simulink model "PHIL_SupportFunctions"  (R2016a)
settings: Solver=FixedStepDiscrete  StartTime=0.0  StopTime=15  FixedStep=1e-2  RelTol=1e-3
settings Model: Creator=CoSES_HPC2  LastModifiedBy=CoSES_HPC2
settings DebuggingCC: RootOutportRequireBusObject=error  StrictBusMsg=ErrorOnBusTreatedAsVector
settings HardwareCC: ProdBitPerPointer=32  ProdLargestAtomicFloat=None  ProdWordSize=32  ProdHWDeviceType=Intel->x86/Pentium
settings RTWCC: SystemTargetFile=NIVeriStand.tlc  TemplateMakefile=NIVeriStand_vc.tmf  Description=NI Phar Lap Real-Time & Windows Targets
settings STFCustomTargetCC: MatFileLogging=on  SystemTargetFile=NIVeriStand.tlc
settings GRTTargetCC: ParMdlRefBuildCompliant=off  CompOptLevelCompliant=off  ConcurrentExecutionCompliant=off  GeneratePreprocessorConditionals=Use local settings  CombineOutputUpdateFcns=off  CPPClassGenCompliant=off  GRTInterface=on  UseToolchainInfoCompliant=off

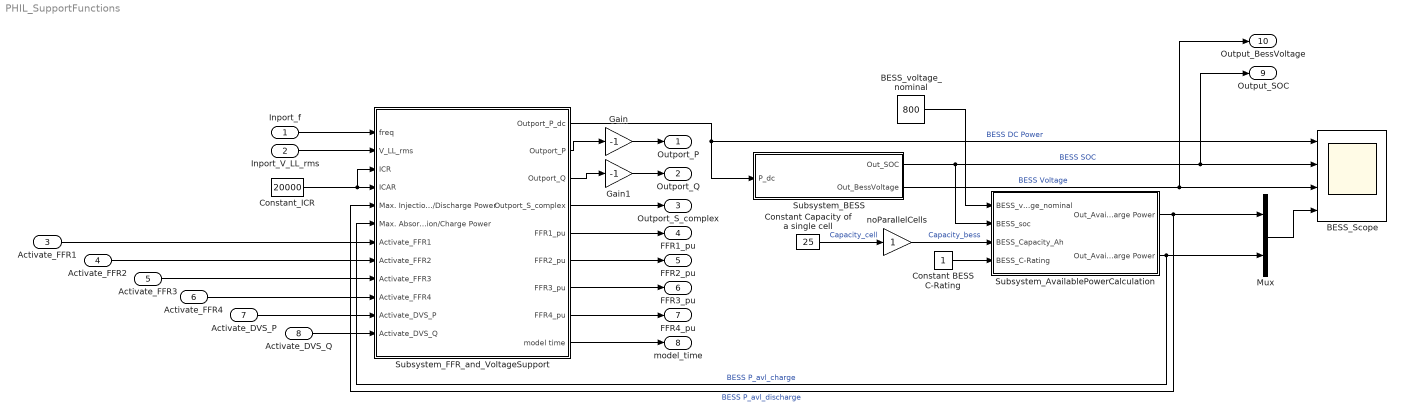
== system PHIL_SupportFunctions ==
  Inport_f : Inport
  Inport_V_LL_rms : Inport  Port=2
  Activate_FFR1 : Inport  Port=3
  Activate_FFR2 : Inport  Port=4
  Activate_FFR3 : Inport  Port=5
  Activate_FFR4 : Inport  Port=6
  Activate_DVS_P : Inport  Port=7
  Activate_DVS_Q : Inport  Port=8
  BESS_Scope : Scope  NumInputPorts=4
  BESS_voltage_nominal : Constant  Value=800
  Constant BESS C-Rating : Constant
  Constant Capacity of a single cell : Constant  Value=25
  Constant_ICR : Constant  Value=20000
  Gain : Gain  Gain=-1
  Gain1 : Gain  Gain=-1
  Mux : Mux  Inputs=2
  Subsystem_AvailablePowerCalculation : Subsystem
  Subsystem_BESS : Subsystem
  Subsystem_FFR_and_VoltageSupport : Subsystem
  noParallelCells : Gain
  Outport_P : Outport
  Outport_Q : Outport  Port=2
  Outport_S_complex : Outport  Port=3
  FFR1_pu : Outport  Port=4
  FFR2_pu : Outport  Port=5
  FFR3_pu : Outport  Port=6
  FFR4_pu : Outport  Port=7
  model_time : Outport  Port=8
  Output_SOC : Outport  Port=9
  Output_BessVoltage : Outport  Port=10
  wires:
  Constant_ICR/1 -> Subsystem_FFR_and_VoltageSupport/3(ICR), Subsystem_FFR_and_VoltageSupport/4(ICAR)
  Subsystem_AvailablePowerCalculation/2(Out_Available Charge Power) -> Subsystem_FFR_and_VoltageSupport/6(Max. Absorption/Charge Power), Mux/2  "BESS P_avl_charge"
  noParallelCells/1 -> Subsystem_AvailablePowerCalculation/3(BESS_Capacity_Ah)  "Capacity_bess"
  Subsystem_BESS/2(Out_BessVoltage) -> Output_BessVoltage/1, BESS_Scope/3  "BESS Voltage"
  Constant BESS C-Rating/1 -> Subsystem_AvailablePowerCalculation/4(BESS_C-Rating)
  Mux/1 -> BESS_Scope/4
  Subsystem_AvailablePowerCalculation/1(Out_Available Discharge Power) -> Subsystem_FFR_and_VoltageSupport/5(Max. Injection/Discharge Power), Mux/1  "BESS P_avl_discharge"
  Subsystem_BESS/1(Out_SOC) -> Output_SOC/1, BESS_Scope/2, Subsystem_AvailablePowerCalculation/2(BESS_soc)  "BESS SOC"
  BESS_voltage_nominal/1 -> Subsystem_AvailablePowerCalculation/1(BESS_voltage_nominal)
  Constant Capacity of a single cell/1 -> noParallelCells/1  "Capacity_cell"
  Subsystem_FFR_and_VoltageSupport/1(Outport_P_dc) -> BESS_Scope/1, Subsystem_BESS/1(P_dc)  "BESS DC Power"
  Subsystem_FFR_and_VoltageSupport/8(FFR4_pu) -> FFR4_pu/1
  Subsystem_FFR_and_VoltageSupport/7(FFR3_pu) -> FFR3_pu/1
  Subsystem_FFR_and_VoltageSupport/6(FFR2_pu) -> FFR2_pu/1
  Subsystem_FFR_and_VoltageSupport/5(FFR1_pu) -> FFR1_pu/1
  Subsystem_FFR_and_VoltageSupport/4(Outport_S_complex) -> Outport_S_complex/1
  Inport_V_LL_rms/1 -> Subsystem_FFR_and_VoltageSupport/2(V_LL_rms)
  Inport_f/1 -> Subsystem_FFR_and_VoltageSupport/1(freq)
  Subsystem_FFR_and_VoltageSupport/9(model time) -> model_time/1
  Gain/1 -> Outport_P/1
  Subsystem_FFR_and_VoltageSupport/2(Outport_P) -> Gain/1
  Gain1/1 -> Outport_Q/1
  Subsystem_FFR_and_VoltageSupport/3(Outport_Q) -> Gain1/1
  Activate_FFR1/1 -> Subsystem_FFR_and_VoltageSupport/7(Activate_FFR1)
  Activate_FFR2/1 -> Subsystem_FFR_and_VoltageSupport/8(Activate_FFR2)
  Activate_FFR3/1 -> Subsystem_FFR_and_VoltageSupport/9(Activate_FFR3)
  Activate_FFR4/1 -> Subsystem_FFR_and_VoltageSupport/10(Activate_FFR4)
  Activate_DVS_P/1 -> Subsystem_FFR_and_VoltageSupport/11(Activate_DVS_P)
  Activate_DVS_Q/1 -> Subsystem_FFR_and_VoltageSupport/12(Activate_DVS_Q)

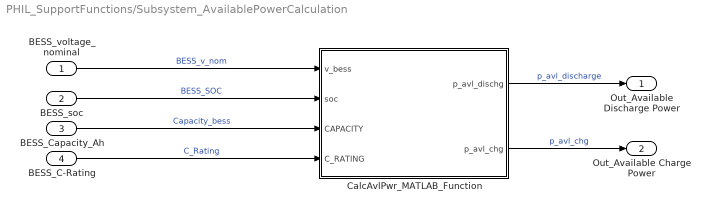
== system PHIL_SupportFunctions/Subsystem_AvailablePowerCalculation ==
  BESS_voltage_nominal : Inport
  BESS_soc : Inport  Port=2
  BESS_Capacity_Ah : Inport  Port=3
  BESS_C-Rating : Inport  Port=4
  CalcAvlPwr_MATLAB_Function : MATLAB Function  TreatAsAtomicUnit=on
  Out_Available Discharge Power : Outport
  Out_Available Charge Power : Outport  Port=2
  wires:
  CalcAvlPwr_MATLAB_Function/1(p_avl_dischg) -> Out_Available Discharge Power/1  "p_avl_discharge"
  BESS_voltage_nominal/1 -> CalcAvlPwr_MATLAB_Function/1(v_bess)  "BESS_v_nom"
  BESS_Capacity_Ah/1 -> CalcAvlPwr_MATLAB_Function/3(CAPACITY)  "Capacity_bess"
  CalcAvlPwr_MATLAB_Function/2(p_avl_chg) -> Out_Available Charge Power/1  "p_avl_chg"
  BESS_soc/1 -> CalcAvlPwr_MATLAB_Function/2(soc)  "BESS_SOC"
  BESS_C-Rating/1 -> CalcAvlPwr_MATLAB_Function/4(C_RATING)  "C_Rating"

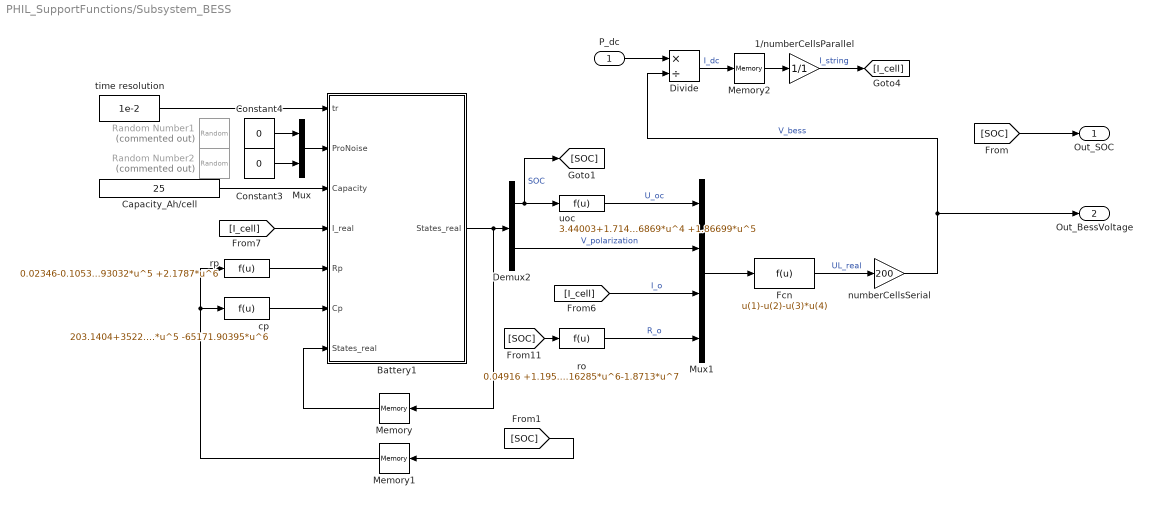
== system PHIL_SupportFunctions/Subsystem_BESS ==
  P_dc : Inport
  1/numberCellsParallel : Gain  Gain=1/1
  Battery1 : MATLAB Function  TreatAsAtomicUnit=on
  Capacity_Ah/cell : Constant  Value=25
  Constant3 : Constant  Value=0
  Constant4 : Constant  Value=0
  Demux2 : Demux  Outputs=2
  Divide : Product  Inputs=*/
  Fcn : Fcn  Expr=u(1)-u(2)-u(3)*u(4)
  Memory : Memory  X0=[0.6;0]  LinearizeAsDelay=on
  Memory1 : Memory  X0=0.6  LinearizeAsDelay=on
  Memory2 : Memory
  Mux : Mux  Inputs=2
  Mux1 : Mux
  Random Number1 : RandomNumber  Commented=on  Variance=2e-8  SampleTime=5e-4
  Random Number2 : RandomNumber  Commented=on  Variance=1e-8  SampleTime=5e-4
  cp : Fcn  Expr=203.1404+3522.78847*u-31392.66753*u^2+122406.91269*u^3-227590.94382*u^4+198281.56406*u^5 -65171.90395*u^6
  numberCellsSerial : Gain  Gain=200
  ro : Fcn  Expr=0.04916 +1.19552*u-6.25333*u^2+14.24181*u^3-13.93388*u^4+2.553*u^5+4.16285*u^6-1.8713*u^7
  rp : Fcn  Expr=0.02346-0.10537*u^1+1.1371*u^2-4.55188*u^3+8.26827*u^4-6.93032*u^5 +2.1787*u^6
  time resolution : Constant  Value=1e-2
  uoc : Fcn  Expr=3.44003+1.71448*u -3.51247*u^2 +5.70868*u^3 -5.06869*u^4 +1.86699*u^5
  Out_SOC : Outport
  Out_BessVoltage : Outport  Port=2
  wires:
  Mux/1 -> Battery1/2(ProNoise)
  Fcn/1 -> numberCellsSerial/1  "UL_real"
  Memory1/1 -> cp/1, rp/1
  time resolution/1 -> Battery1/1(tr)
  Memory/1 -> Battery1/7("States_real ")
  ro/1 -> Mux1/4  "R_o"
  uoc/1 -> Mux1/1  "U_oc"
  Demux2/1 -> [SOC], uoc/1  "SOC"
  Demux2/2 -> Mux1/2  "V_polarization"
  Mux1/1 -> Fcn/1
  Constant3/1 -> Mux/2
  Constant4/1 -> Mux/1
  [I_cell] -> Mux1/3  "I_o"
  Battery1/1(States_real) -> Memory/1, Demux2/1
  rp/1 -> Battery1/5(Rp)
  cp/1 -> Battery1/6(Cp)
  Capacity_Ah/cell/1 -> Battery1/3(Capacity)
  P_dc/1 -> Divide/1
  Divide/1 -> Memory2/1  "I_dc"
  Memory2/1 -> 1/numberCellsParallel/1
  [I_cell] -> Battery1/4(I_real)
  1/numberCellsParallel/1 -> [I_cell]  "I_string"
  numberCellsSerial/1 -> Divide/2, Out_BessVoltage/1  "V_bess"
  [SOC] -> Out_SOC/1
  [SOC] -> Memory1/1
  [SOC] -> ro/1

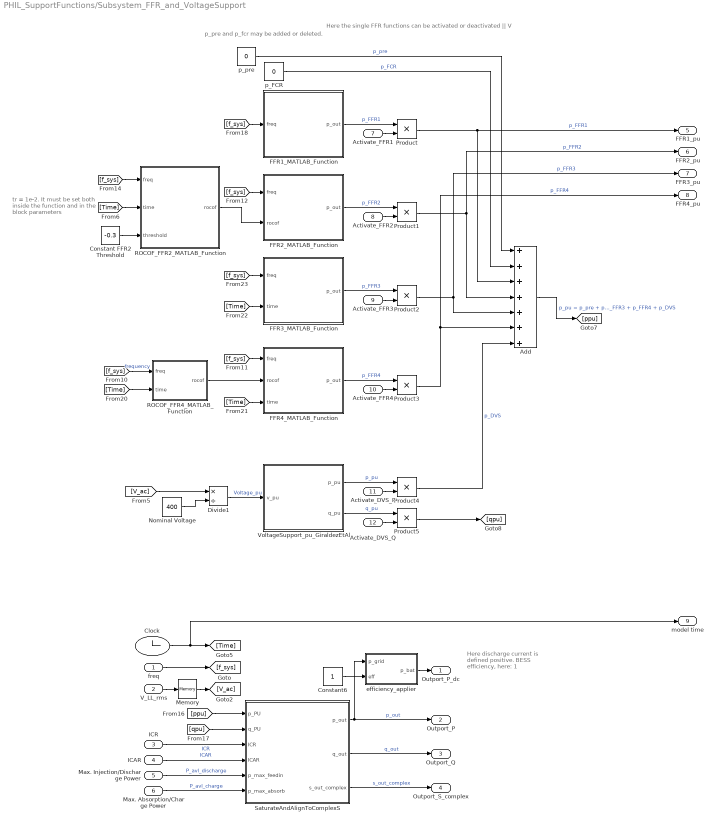
== system PHIL_SupportFunctions/Subsystem_FFR_and_VoltageSupport ==
  note: tr = 1e-2. It must be set
      | both inside the function
      | and in the block parameters
  note: Here discharge
      | current is defined positive.
      | BESS efficiency, here: 1
  note: Here the single FFR functions can be activated or deactivated
      |                                                ||
      |                                                V
  note: p_pre and p_fcr may be added or deleted.
  freq : Inport
  V_LL_rms : Inport  Port=2
  ICR : Inport  Port=3
  ICAR : Inport  Port=4
  Max. Injection/Discharge Power : Inport  Port=5
  Max. Absorption/Charge Power : Inport  Port=6
  Activate_FFR1 : Inport  Port=7
  Activate_FFR2 : Inport  Port=8
  Activate_FFR3 : Inport  Port=9
  Activate_FFR4 : Inport  Port=10
  Activate_DVS_P : Inport  Port=11
  Activate_DVS_Q : Inport  Port=12
  Add : Sum  Inputs=+++++++
  Clock : Clock
  Constant FFR2 Threshold : Constant  Value=-0.3
  Constant6 : Constant
  Divide1 : Product  Inputs=*/
  FFR1_MATLAB_Function : MATLAB Function  TreatAsAtomicUnit=on  SystemSampleTime=1e-2
  FFR2_MATLAB_Function : MATLAB Function  TreatAsAtomicUnit=on  SystemSampleTime=1e-2
  FFR3_MATLAB_Function : MATLAB Function  TreatAsAtomicUnit=on  SystemSampleTime=1e-2
  FFR4_MATLAB_Function : MATLAB Function  TreatAsAtomicUnit=on  SystemSampleTime=1e-2
  Memory : Memory  X0=400
  Nominal Voltage : Constant  Value=400
  Product{,1..5} (6 alike) : Product
  ROCOF_FFR2_MATLAB_Function : MATLAB Function  TreatAsAtomicUnit=on  SystemSampleTime=1e-2
  ROCOF_FFR4_MATLAB_Function : MATLAB Function  TreatAsAtomicUnit=on  SystemSampleTime=1e-2
  SaturateAndAlignToComplexS : MATLAB Function  TreatAsAtomicUnit=on
  VoltageSupport_pu_GiraldezEtAl : MATLAB Function  TreatAsAtomicUnit=on
  efficiency_applier : MATLAB Function  TreatAsAtomicUnit=on
  p_FCR : Constant  Value=0
  p_pre : Constant  Value=0
  Outport_P_dc : Outport
  Outport_P : Outport  Port=2
  Outport_Q : Outport  Port=3
  Outport_S_complex : Outport  Port=4
  FFR1_pu : Outport  Port=5
  FFR2_pu : Outport  Port=6
  FFR3_pu : Outport  Port=7
  FFR4_pu : Outport  Port=8
  model time : Outport  Port=9
  wires:
  efficiency_applier/1(p_bat) -> Outport_P_dc/1
  freq/1 -> [f_sys]
  Max. Injection/Discharge Power/1 -> SaturateAndAlignToComplexS/5(p_max_feedin)  "P_avl_discharge"
  Nominal Voltage/1 -> Divide1/2
  Divide1/1 -> VoltageSupport_pu_GiraldezEtAl/1(v_pu)  "Voltage_pu"
  Max. Absorption/Charge Power/1 -> SaturateAndAlignToComplexS/6(p_max_absorb)  "P_avl_charge"
  SaturateAndAlignToComplexS/2(q_out) -> Outport_Q/1  "q_out"
  SaturateAndAlignToComplexS/3(s_out_complex) -> Outport_S_complex/1  "s_out_complex"
  Memory/1 -> [V_ac]
  [ppu] -> SaturateAndAlignToComplexS/1(p_PU)
  [qpu] -> SaturateAndAlignToComplexS/2(q_PU)
  SaturateAndAlignToComplexS/1(p_out) -> efficiency_applier/1(p_grid), Outport_P/1  "p_out"
  ICR/1 -> SaturateAndAlignToComplexS/3(ICR)  "ICR"
  ICAR/1 -> SaturateAndAlignToComplexS/4(ICAR)  "ICAR"
  Product5/1 -> [qpu]
  Product/1 -> Add/3, FFR1_pu/1  "p_FFR1"
  ROCOF_FFR4_MATLAB_Function/1(rocof) -> FFR4_MATLAB_Function/2(rocof)
  FFR2_MATLAB_Function/1(p_out) -> Product1/1  "p_FFR2"
  ROCOF_FFR2_MATLAB_Function/1(rocof) -> FFR2_MATLAB_Function/2(rocof)
  p_FCR/1 -> Add/2  "p_FCR"
  Product3/1 -> FFR4_pu/1, Add/6  "p_FFR4"
  [f_sys] -> FFR3_MATLAB_Function/1(freq)
  FFR1_MATLAB_Function/1(p_out) -> Product/1  "p_FFR1"
  p_pre/1 -> Add/1  "p_pre"
  FFR4_MATLAB_Function/1(p_out) -> Product3/1  "p_FFR4"
  [f_sys] -> FFR2_MATLAB_Function/1(freq)
  FFR3_MATLAB_Function/1(p_out) -> Product2/1  "p_FFR3"
  [f_sys] -> ROCOF_FFR2_MATLAB_Function/1(freq)
  [Time] -> FFR3_MATLAB_Function/2(time)
  Constant FFR2 Threshold/1 -> ROCOF_FFR2_MATLAB_Function/3(threshold)
  Product1/1 -> Add/4, FFR2_pu/1  "p_FFR2"
  Product2/1 -> FFR3_pu/1, Add/5  "p_FFR3"
  Clock/1 -> model time/1, [Time]
  [f_sys] -> ROCOF_FFR4_MATLAB_Function/1(freq)  "frequency"
  [f_sys] -> FFR4_MATLAB_Function/1(freq)
  [Time] -> FFR4_MATLAB_Function/3(time)
  [Time] -> ROCOF_FFR4_MATLAB_Function/2(time)
  [f_sys] -> FFR1_MATLAB_Function/1(freq)
  [Time] -> ROCOF_FFR2_MATLAB_Function/2(time)
  Product4/1 -> Add/7  "p_DVS"
  Add/1 -> [ppu]  "p_pu = p_pre + p_FFR1 + p_FFR2 + p_FFR3 + p_FFR4 + p_DVS"
  VoltageSupport_pu_GiraldezEtAl/2(q_pu) -> Product5/1  "q_pu"
  VoltageSupport_pu_GiraldezEtAl/1(p_pu) -> Product4/1  "p_pu"
  V_LL_rms/1 -> Memory/1
  Activate_FFR1/1 -> Product/2
  Activate_FFR3/1 -> Product2/2
  Activate_FFR2/1 -> Product1/2
  Activate_FFR4/1 -> Product3/2
  Activate_DVS_P/1 -> Product4/2
  Activate_DVS_Q/1 -> Product5/2
  [V_ac] -> Divide1/1
  Constant6/1 -> efficiency_applier/2(eff)

== matlab function PHIL_SupportFunctions/Subsystem_FFR_and_VoltageSupport/SaturateAndAlignToComplexS ==
  data: p_out output; q_out output; p_PU input; q_PU input; s_out_complex output; ICR input; ICAR input; p_max_feedin input; p_max_absorb input
% This function computes the complex power reference for the converter from
% the p.u. values of active and reactive power, respectively, as well as
% the maximum converter power and the maximum available BESS power.
%
% Active power is defined as positive when supplying energy to the grid (=discharging the BESS)
%
%##### Input description #####
% p_PU         : active power reference (in p.u.)
% q_PU         : reactive power reference (in p.u.)
% ICR          : Maximum Converter Power (in VA) (ICR = IBR continuous rating, IBR = Inverter-Based Resources)
% ICAR         : Maximum Converter Power for absorption (in VA) (ICAR = IBR continuous absorption rating)
% p_max_feedin : Maximum available Power from BESS for feedin / discharge BESS (in W)
% p_max_absorb : Maximum available Power from BESS for absorption / charge BESS (in W)
%##### Output description #####
% p_out        : Active Power Reference (in W)
% q_out        : Reactive Power Reference (in var)
% s_out_complex: Complex Power Reference (in VA)

function [p_out,q_out,s_out_complex]  = ComplexApparentPower(p_PU, q_PU, ICR, ICAR, p_max_feedin, p_max_absorb)
% ISR in Watt (ISR = IBR short-term rating) may be added

% Reactive Power
q_out = q_PU*ICR; % q_PU is already saturated to +-0.44, hence no further treatment necessary

% Active Power
if p_PU >= 1              % positive active power, Saturation and Limiting to maximum grid injection / BESS discharge power
    p_out = p_max_feedin; 
elseif p_PU > 0           % positive active power, linear FFR range
    p_out = p_PU * p_max_feedin;
elseif p_PU <= -1         % negative active power, Saturation and Limiting to maximum grid absorption / BESS charge power
    p_out = -abs(p_max_absorb); 
elseif p_PU < 0           % negative active power, linear Voltage support range
    p_out = p_PU * abs(p_max_absorb); % (p_pu is already negative, so multiply with a positive number)
else % p_PU == 0          % zero output power
    p_out = 0;
end

% Complex Power
s_out_complex = complex(p_out,q_out); 
if p_out < 0
    if abs(s_out_complex) > ICAR
        p_out = -sqrt((ICAR^2)-(q_out^2));
    end
else % p_out >= 0
    if abs(s_out_complex) > ICR
        p_out = sqrt((ICR^2)-(q_out^2));
    end
end
    s_out_complex = complex(p_out,q_out); 
end

== matlab function PHIL_SupportFunctions/Subsystem_FFR_and_VoltageSupport/VoltageSupport_pu_GiraldezEtAl ==
  data: v_pu input; p_pu output; q_pu output
% This function computes the active and reactive output power in p.u. from
% the measured grid voltage in p.u. according to [Giraldez et al.]

function [p_pu,q_pu] = VoltageSupport(v_pu)

Q_max = 0.44; % in p.u.

if v_pu >= 0.97 && v_pu <= 1.03
    p_pu = 0;
    q_pu = 0;
elseif v_pu > 1.03
    if v_pu < 1.06
        p_pu = 0;
        q_pu = (1.03-v_pu)*(Q_max/0.03);
    elseif v_pu < 1.1
        p_pu = (1.06-v_pu)*(1/0.04);
        q_pu = -Q_max;
    else % v_pu >= 1.1
        p_pu = -1;
        q_pu = -Q_max;
    end
else % v_pu < 0.97
    p_pu = 0;
    if v_pu > 0.94
        q_pu = (0.97-v_pu)*(Q_max/0.03);
    else % v_pu <= 0.94
        q_pu = Q_max;
    end
end
end

== matlab function PHIL_SupportFunctions/Subsystem_AvailablePowerCalculation/CalcAvlPwr_MATLAB_Function ==
  data: v_bess input; p_avl_dischg output; soc input; CAPACITY input; p_avl_chg output; C_RATING input
% This function computes the Battery Energy Storage's (BESS') 
% available power for both the discharging and charging case.
% 
%##### Input description #####
% v_bess  : Voltage (V) of the BESS
% soc     : State of Charge (p.u. (1 means full)) of the BESS
% CAPACITY: Capacity (Ah) of the BESS
% C_RATING: C-Rating (p.u.) of the BESS = of the cells
%##### Output description #####
% p_avl_dischg: maximum available discharge power (W) 
% p_avl_chg   : maximum available charge power (W)

function [p_avl_dischg,p_avl_chg] = CalcAvailablePwr(v_bess, soc, CAPACITY, C_RATING) 
%% Constants Definition
DERATING_START_AT_SOC = 0.3;    % Assuming linear derating from SOC=30% downwards and from 70% upwards
P_MAX = C_RATING * CAPACITY * v_bess;  % Maximum BESS power, w/o consideration of SOC.

%% Algorithm for Calculation of available Discharge Power
if soc > DERATING_START_AT_SOC
    p_avl_dischg = P_MAX;
elseif soc > 0
    p_avl_dischg = P_MAX * soc / DERATING_START_AT_SOC;
else 
    p_avl_dischg = 0;
end

%% Algorithm for Calculation of available Charge Power
if soc < (1-DERATING_START_AT_SOC)
    p_avl_chg = P_MAX;
elseif soc < 1
    p_avl_chg = P_MAX * (1-soc) / DERATING_START_AT_SOC;
else
    p_avl_chg = 0;
end
end

== matlab function PHIL_SupportFunctions/Subsystem_FFR_and_VoltageSupport/FFR1_MATLAB_Function ==
  data: freq input; p_out output
% This function computes the FFR_1 power output in p.u. based on the
% current measured or observed frequency handed over in Hz. 

function p_out = FFR_1(freq)

fnom = 50;       % 50 Hz
fUF_FFR1 = 49.9; % Minimum: 99.17% of fnom, Maximum: 99.94% of fnom, Default: 99.94% of fnom [IEEE Std 2800-2022], Here: 99.8% of fnom
kUF_FFR1 = 0.01; % Minimum: 1%, Maximum: 5%, Default: 1% [IEEE Std 2800-2022]

if freq<fUF_FFR1
    p_out = (fUF_FFR1 - freq)/(fnom*kUF_FFR1);
else
    p_out = 0;
end
end

== matlab function PHIL_SupportFunctions/Subsystem_FFR_and_VoltageSupport/FFR2_MATLAB_Function ==
  data: freq input; p_out output; rocof input
% This function computes the FFR_2 power output in p.u. based on the
% current frequency in Hz and rate of change of frequency (RoCoF) in Hz/s, 
% both handed over as transfer parameters.

function p_out = FFR_2(freq, rocof)

fnom = 50;       % 50 Hz (here just informative)
fUF_FFR2 = 49.7; % Min: 99.17% of fnom, Max: N/A, Default: 99.4% of fnom (used here) [IEEE Std 2800-2022]
kUF_FFR2 = 0.5;  % Min: 0, Max: 5, Default: 0.5 [IEEE Std 2800-2022], (Here: 2.5)

if freq>fUF_FFR2 % idle, i.e. NOT triggered
    p_out = 0;
else % triggered, i.e. freq <= fUF_FFR2
    p_out = -kUF_FFR2 * rocof;
end
end

== matlab function PHIL_SupportFunctions/Subsystem_FFR_and_VoltageSupport/FFR4_MATLAB_Function ==
  data: freq input; rocof input; p_out output; time input
% This function computes the FFR_4 power output in p.u. based on passed
% frequency in Hz, rate of change of frequency (RoCoF) in Hz/s and time 
% in seconds. All three are handed over as transfer parameters. 

function p_out = FFR_4(freq, rocof, time)

fnom = 50;           % 50 Hz
dtrigUF_FFR4 = -0.1; % Min: -5.0 Hz/s, Max: 0 Hz/s, Default: -0,5 Hz/s [IEEE Std 2800-2022], Here: -0.1 Hz/s
pT4UF_FFR4 = 0.1;    % Min: 0 p.u., Max: 1 p.u., Default: 0.1 p.u. [IEEE Std 2800-2022], Here: 0.1 p.u.

t_holdFFR = 30;      % [IEEE Std 2800-2022], Annex K.3 (time to hold the support when the trigger is not active any more but frequency has not reached fnom yet)
t_rampFFR = 300;     % [IEEE Std 2800-2022], Annex K.4 (time to ramp down the support after t_holdFFR has been exceeded and fnom has not been reached yet) 

persistent t_trigger;
if isempty(t_trigger)
    t_trigger = -999;
end

if freq<=fnom
    if rocof<=dtrigUF_FFR4 % TRIGGER  (greater/less sign swapped compared to [IEEE Std 2800-2022])
        t_trigger = time; % may be set several times, stores the last trigger event
        p_out = pT4UF_FFR4;
    else % (rocof > dtrigUF_FFR4) AND freq <= fnom: continue operation during t_holdFFR and derate for t_rampFFR
        if (time - t_trigger) <= t_holdFFR % continue
            p_out = pT4UF_FFR4; 
        elseif (time - t_trigger) <= (t_holdFFR+t_rampFFR) % derate
            p_out = pT4UF_FFR4*(1-(time - t_trigger - t_holdFFR) / (t_rampFFR)); 
        else % time elapsed since last trigger event > (t_holdFFR+t_rampFFR)
            p_out = 0;
        end
    end
else % freq>fnom
    t_trigger = -999; % reset trigger
    p_out = 0; 
end
end

== matlab function PHIL_SupportFunctions/Subsystem_FFR_and_VoltageSupport/FFR3_MATLAB_Function ==
  data: freq input; p_out output; time input
% This function computes the FFR_3 power output in p.u. based on the
% current frequency in Hz and time in seconds. Both are handed over as
% transfer parameters.

function p_out = FFR_3(freq, time)

fnom = 50;            % 50 Hz
fUF_FFR3 = 49.7;      % basic support threshold (where pT3UF_FFR3 is used)
fUF_FFR3_1 = 49.65;   % 1st extra support threshold (where pT3UF_FFR3_1 is used)
fUF_FFR3_2 = 49.6;    % 2nd extra support threshold (where pT3UF_FFR3_2 is used)
pT3UF_FFR3 = 0.33;    % basic support power
pT3UF_FFR3_1 = 0.66;  % 1st extra support power
pT3UF_FFR3_2 = 1;     % 2nd extra support power
t_holdFFR = 30;       % [IEEE Std 2800-2022], Annex K.3 (time to hold the support when the trigger is not active any more but frequency has not reached fnom yet)
t_rampFFR = 300;      % [IEEE Std 2800-2022], Annex K.4 (time to ramp down the support after t_holdFFR has been exceeded and fnom has not been reached yet) 

persistent t_trigger;
if isempty(t_trigger)
    t_trigger = -999;
end

if freq<=fnom
    if freq>fUF_FFR3_1     % freq=(fUF_FFR3_1 , fUF_FFR3]
        P = pT3UF_FFR3;
    elseif freq>fUF_FFR3_2 % freq=(fUF_FFR3_2 , fUF_FFR3_1]
        P = pT3UF_FFR3_1;
    elseif freq>=47.5      % freq=[47.5 , fUF_FFR3_2]
        P = pT3UF_FFR3_2;
    else                   % freq<47.5 Hz
        P = 0;
    end

    if freq<fUF_FFR3 % Trigger
        t_trigger = time; % may be set several times, stores last trigger event
        p_out = P;
    else % fUF_FFR3 <= freq <= fnom: continue operation during t_holdFFR and derate for t_rampFFR
        if (time - t_trigger) <= t_holdFFR % hold
            p_out = P;
        elseif (time - t_trigger) <= (t_holdFFR+t_rampFFR) % derate
            p_out = P*(1-(time - t_trigger - t_holdFFR) / (t_rampFFR));
        else % time elapsed since last trigger event > (t_holdFFR+t_rampFFR)
            p_out = 0;
        end
    end

else % freq>fnom
    t_trigger = -999; % reset trigger
    p_out = 0;
end
end

== matlab function PHIL_SupportFunctions/Subsystem_FFR_and_VoltageSupport/ROCOF_FFR2_MATLAB_Function ==
  data: freq input; rocof output; time input; threshold input
% This function computes the rate of change of frequency (RoCoF) over a
% 500ms window only after it has been triggered by the incremental df/dt
% being below or equal to the transfer parameter "threshold". 
% The particular RoCoF will be returned for 30 seconds and return zeros 
% until it is triggered again.
%
%##### Input description #####
% freq     : freqency input (Hz)
% time     : time input (s)
% threshold: for triggering the rocof calculation over 500ms shall be negative and in Hz/s
% tr       : must be the same as the time resolution of the simulation, i.e. step size (typ. 0.1s, max. 0.5s).
%##### Output description #####
% rocof: standard output is zero. After the incremental difference df/dt falls
%        below the threshold value, the algorithm starts calculating the
%        rocof over a 0.5s window and outputs it as soon as available.

function rocof = ROCOF_FFR2(freq, time, threshold) 
%% Definition of persistent variables
tr = 1e-2;
persistent fcurrent;
if isempty(fcurrent)
    fcurrent = freq;
end

persistent tcurrent;
if isempty(tcurrent)
    tcurrent = -1;
end

persistent fminus1;
persistent tminus1;

persistent isTriggered;
if isempty(isTriggered)
    isTriggered = false;
end

persistent tTriggered;
if isempty(tTriggered)
    tTriggered=-31;
end

persistent rollingWindow;
if isempty(rollingWindow)
    rollingWindow = zeros(0.5/tr,2); % Creating the rolling window with 2 columns and 0.5s/tr rows, e.g. for tr=0.1s 5 rows
end

%% Start of algorithm
    tminus1 = tcurrent;
    tcurrent = time;
    fminus1 = fcurrent;
    fcurrent = freq;

    if isTriggered == false % Incremental difference one step until triggered
        rocof = 0;

        df = fcurrent-fminus1;
        dt = tcurrent-tminus1;
        dfdt = df/dt;
    
        if dfdt <= threshold
            isTriggered = true;
            tTriggered = tminus1;
            rollingWindow(1,:)=[tminus1,fminus1];
            rollingWindow(2,:)=[tcurrent,fcurrent];
        end
    else % isTriggered == true
        if (tcurrent-tTriggered) >= 29.9999 % cannot use ">= 30" due to limited exactness
            isTriggered = false;
            rocof = 0;
        elseif (tcurrent-tTriggered) >= 0.4999 % cannot use ">= 0.5" due to limited exactness
            fminus500ms = rollingWindow(mod((round((tcurrent-0.5-tTriggered)/tr)),round(0.5/tr))+1,2);
            rocof = (fcurrent - fminus500ms)/0.5; % calculate rocof over a 0.5s = 500ms window
            % store the current time and frequency values
            rollingWindow(mod((round((tcurrent-0.5-tTriggered)/tr)),round(0.5/tr))+1,:) = [tcurrent,fcurrent];
        else % (tcurrent-tTriggered) < 0.5
            rocof = 0; % ride-through for the first 500 ms after trigger event, i.e. before the rolling window is operable
            % store the current time and frequency values
            rollingWindow((round((tcurrent-tTriggered)/tr))+1,:) = [tcurrent,fcurrent];
        end
    end
end

== matlab function PHIL_SupportFunctions/Subsystem_FFR_and_VoltageSupport/ROCOF_FFR4_MATLAB_Function ==
  data: freq input; rocof output; time input
% This function computes the rate of change of frequency (RoCoF) in Hz/s 
% of one sample based on the previous sample. 
% 
%##### Input description #####
% freq: freqency input (Hz)
% time: time input (seconds)
%##### Output description #####
% rocof: Output is the derivative of freq, i.e. the quotient of the
% difference between the current and previous step in frequency and time: 
% delta_f/delta_t.

function rocof = ROCOF_FFR4(freq, time) 
%% Definition of persistent variables
persistent fcurrent;
if isempty(fcurrent)
    fcurrent = freq;
end

persistent tcurrent;
if isempty(tcurrent)
    tcurrent = -1;
end

persistent fminus1;
persistent tminus1;
%% Start of algorithm
    tminus1 = tcurrent;
    tcurrent = time;
    fminus1 = fcurrent;
    fcurrent = freq;

    % Incremental difference one step until triggered
    delta_f = fcurrent-fminus1;
    delta_t = tcurrent-tminus1;
    rocof = delta_f/delta_t;
end

== matlab function PHIL_SupportFunctions/Subsystem_BESS/Battery1 ==
  settings: updateMethod=DISCRETE
  data: tr input; States_real output; ProNoise input; Capacity input; I_real input; Rp input; Cp input; States_real input
function States_real = StatReal(tr, ProNoise, Capacity, I_real, Rp, Cp, States_real)
    tao = Rp * Cp;
    Qs = ProNoise(1);
    Qu = ProNoise(2);
    
    A2=exp(-tr/tao);
    A=[1 0;0 A2];  % State transformation matrix
    B1 = -tr/(Capacity*3600);
    B2=Rp*(1-exp(-tr/tao));  
    B=[B1;B2];  % Input control matrix
    States_real = A*States_real + B*I_real + [Qs;Qu];  % 实际过程模拟以 0.1s 更新一次 => Die eigentliche Prozesssimulation wird in 0,1s aktualisiert.

== matlab function PHIL_SupportFunctions/Subsystem_FFR_and_VoltageSupport/efficiency_applier ==
  data: p_grid input; p_bat output; eff input
% This function applies an assumed efficiency of the overall BESS to the
% power that is charged or discharged. I.e. increasing the discharge power
% and decreasing the charged power due to losses.
% 
% >Discharge current is defined positive<
%
%##### Input description #####
% p_grid       : active power drawn from or supplied from the grid (in W)
% eff          : efficiency (0...1)
%
%##### Output description #####
% p_bat        : Active Power drawn from of supplied to ideal storage (in W)


function p_bat = efficiency(p_grid, eff)
if p_grid > 0
    p_bat = p_grid / eff;
elseif p_grid < 0
    p_bat = p_grid * eff;
else
    p_bat = 0;
end
end
